simulink model "th_discrete_time_integrator"  (R2020b)
settings: Solver=VariableStepAuto  StartTime=0.0  StopTime=6  RelTol=1e-3
values from neighbouring files (symbols this model uses):
  parInitCondInitVal = 0.0    [dd_discrete_time_integrator.sldd]
  parInpInitVal = 0.0    [dd_discrete_time_integrator.sldd]
  parIntgGain = 1.0    [dd_discrete_time_integrator.sldd]
  parLowLimInitVal = 0.0    [dd_discrete_time_integrator.sldd]
  parOutpDataTypeInhrFlag = 1    [dd_discrete_time_integrator.sldd]
  parRsetCondInitVal = 0.0    [dd_discrete_time_integrator.sldd]
  parSampTime = 0.01    [dd_discrete_time_integrator.sldd]
  parSatFlag = 0.0    [dd_discrete_time_integrator.sldd]
  parTestProcInitCondIndx = 0.0    [dd_discrete_time_integrator.sldd]
  parTestProcInpIndx = 1.0    [dd_discrete_time_integrator.sldd]
  parTestProcLowLimIndx = 0.0    [dd_discrete_time_integrator.sldd]
  parTestProcRsetCondIndx = 0.0    [dd_discrete_time_integrator.sldd]
  parTestProcUpLimIndx = 0.0    [dd_discrete_time_integrator.sldd]
  parUpLimInitVal = 0.0    [dd_discrete_time_integrator.sldd]
undefined symbols (not defined in the file or in its folder): DiscIntNeverNeededParam
settings Model: DataDictionary=dd_discrete_time_integrator.sldd  Creator=CAV2OFO  LastModifiedBy=CAV2OFO
settings DebuggingCC: SFUnusedDataAndEventsDiag=none

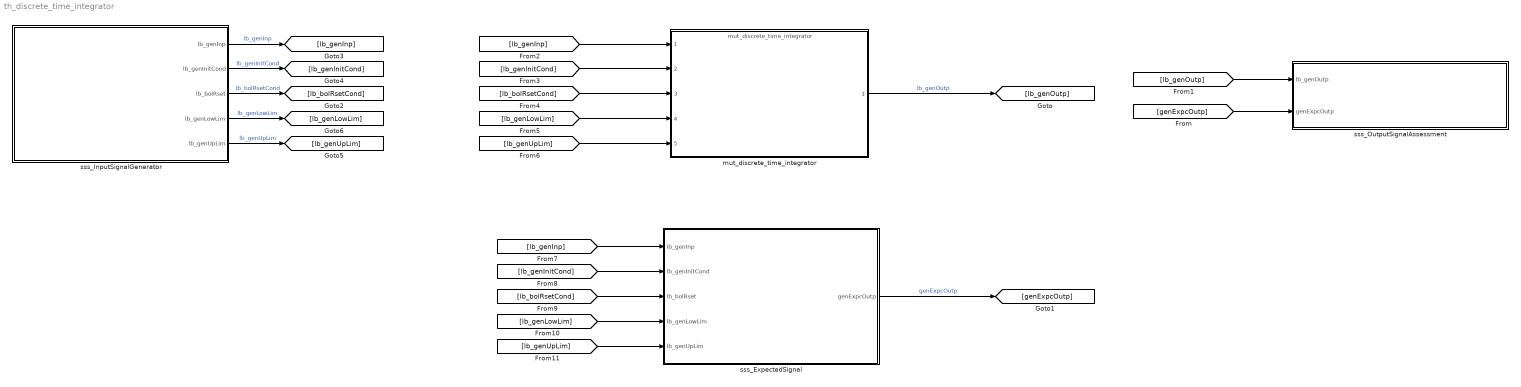
== system th_discrete_time_integrator ==
  mut_discrete_time_integrator : ModelReference  ModelNameDialog=mut_discrete_time_integrator  SimulationMode=Normal  ModelReferenceVersion=1.22
  sss_ExpectedSignal : Subsystem
  sss_InputSignalGenerator : Subsystem
  sss_OutputSignalAssessment : Subsystem
  wires:
  [lb_genUpLim] -> mut_discrete_time_integrator/5
  [lb_genInitCond] -> sss_ExpectedSignal/2(lb_genInitCond)
  sss_InputSignalGenerator/1(lb_genInp) -> [lb_genInp]  "lb_genInp"
  mut_discrete_time_integrator/1 -> [lb_genOutp]  "lb_genOutp"
  [lb_bolRsetCond] -> sss_ExpectedSignal/3(lb_bolRset)
  [lb_genOutp] -> sss_OutputSignalAssessment/1(lb_genOutp)
  [lb_genInitCond] -> mut_discrete_time_integrator/2
  sss_InputSignalGenerator/5(lb_genUpLim) -> [lb_genUpLim]  "lb_genUpLim"
  [genExpcOutp] -> sss_OutputSignalAssessment/2(genExpcOutp)
  [lb_genLowLim] -> sss_ExpectedSignal/4(lb_genLowLim)
  sss_InputSignalGenerator/4(lb_genLowLim) -> [lb_genLowLim]  "lb_genLowLim"
  [lb_bolRsetCond] -> mut_discrete_time_integrator/3
  sss_InputSignalGenerator/2(lb_genInitCond) -> [lb_genInitCond]  "lb_genInitCond"
  [lb_genUpLim] -> sss_ExpectedSignal/5(lb_genUpLim)
  sss_InputSignalGenerator/3(lb_bolRset) -> [lb_bolRsetCond]  "lb_bolRsetCond"
  sss_ExpectedSignal/1(genExpcOutp) -> [genExpcOutp]  "genExpcOutp"
  [lb_genInp] -> sss_ExpectedSignal/1(lb_genInp)
  [lb_genInp] -> mut_discrete_time_integrator/1
  [lb_genLowLim] -> mut_discrete_time_integrator/4

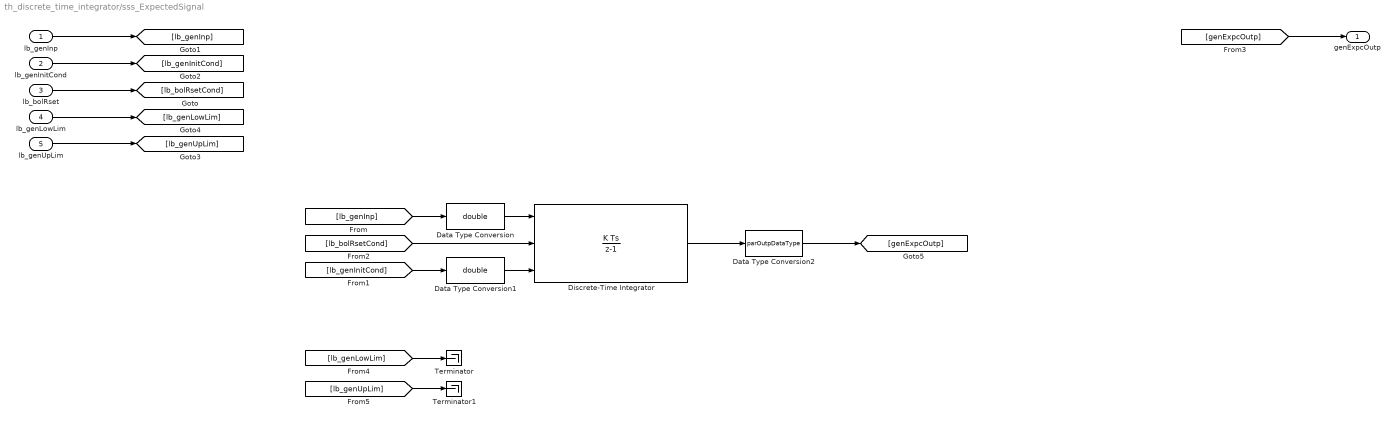
== system th_discrete_time_integrator/sss_ExpectedSignal ==
  lb_genInp : Inport
  lb_genInitCond : Inport  Port=2
  lb_bolRset : Inport  Port=3
  lb_genLowLim : Inport  Port=4
  lb_genUpLim : Inport  Port=5
  Data Type Conversion : DataTypeConversion  OutDataTypeStr=double
  Data Type Conversion1 : DataTypeConversion  OutDataTypeStr=double
  Data Type Conversion2 : DataTypeConversion  OutDataTypeStr=parOutpDataType
  Discrete-Time Integrator : DiscreteIntegrator  gainval=double(parIntgGain)  ExternalReset=level  InitialConditionSource=external  SampleTime=double(parSampTime)  LimitOutput=on  UpperSaturationLimit=double(parUpLimInitVal)  LowerSaturationLimit=double(parLowLimInitVal)  ICPrevOutput=DiscIntNeverNeededParam  ICPrevScaledInput=DiscIntNeverNeededParam
  Terminator : Terminator
  Terminator1 : Terminator
  genExpcOutp : Outport
  wires:
  lb_bolRset/1 -> [lb_bolRsetCond]
  lb_genInp/1 -> [lb_genInp]
  lb_genInitCond/1 -> [lb_genInitCond]
  lb_genLowLim/1 -> [lb_genLowLim]
  lb_genUpLim/1 -> [lb_genUpLim]
  [lb_bolRsetCond] -> Discrete-Time Integrator/2
  [genExpcOutp] -> genExpcOutp/1
  Discrete-Time Integrator/1 -> Data Type Conversion2/1
  [lb_genInitCond] -> Data Type Conversion1/1
  [lb_genInp] -> Data Type Conversion/1
  Data Type Conversion1/1 -> Discrete-Time Integrator/3
  Data Type Conversion2/1 -> [genExpcOutp]
  Data Type Conversion/1 -> Discrete-Time Integrator/1
  [lb_genLowLim] -> Terminator/1
  [lb_genUpLim] -> Terminator1/1

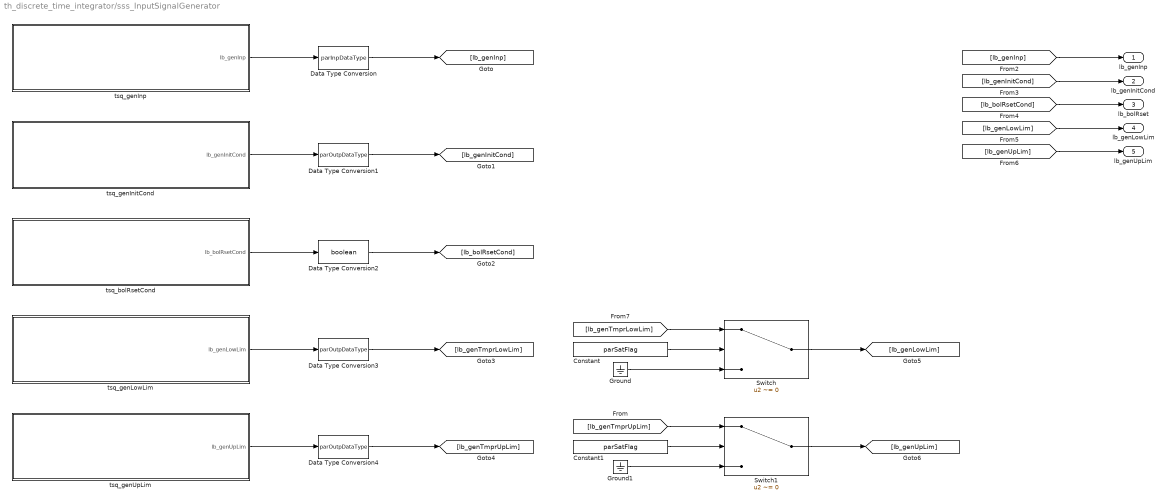
== system th_discrete_time_integrator/sss_InputSignalGenerator ==
  Constant : Constant  Value=parSatFlag
  Constant1 : Constant  Value=parSatFlag
  Data Type Conversion : DataTypeConversion  OutDataTypeStr=parInpDataType
  Data Type Conversion1 : DataTypeConversion  OutDataTypeStr=parOutpDataType
  Data Type Conversion2 : DataTypeConversion  OutDataTypeStr=boolean
  Data Type Conversion3 : DataTypeConversion  OutDataTypeStr=parOutpDataType
  Data Type Conversion4 : DataTypeConversion  OutDataTypeStr=parOutpDataType
  Ground : Ground
  Ground1 : Ground
  Switch : Switch  Criteria=u2 ~= 0
  Switch1 : Switch  Criteria=u2 ~= 0
  tsq_bolRsetCond : Test Sequence  TreatAsAtomicUnit=on
  tsq_genInitCond : Test Sequence  TreatAsAtomicUnit=on
  tsq_genInp : Test Sequence  TreatAsAtomicUnit=on
  tsq_genLowLim : Test Sequence  TreatAsAtomicUnit=on
  tsq_genUpLim : Test Sequence  TreatAsAtomicUnit=on
  lb_genInp : Outport
  lb_genInitCond : Outport  Port=2
  lb_bolRset : Outport  Port=3
  lb_genLowLim : Outport  Port=4
  lb_genUpLim : Outport  Port=5
  wires:
  [lb_genInitCond] -> lb_genInitCond/1
  [lb_genInp] -> lb_genInp/1
  [lb_bolRsetCond] -> lb_bolRset/1
  [lb_genLowLim] -> lb_genLowLim/1
  [lb_genUpLim] -> lb_genUpLim/1
  tsq_genInp/1(lb_genInp) -> Data Type Conversion/1
  Data Type Conversion/1 -> [lb_genInp]
  Data Type Conversion1/1 -> [lb_genInitCond]
  tsq_genInitCond/1(lb_genInitCond) -> Data Type Conversion1/1
  Data Type Conversion2/1 -> [lb_bolRsetCond]
  tsq_bolRsetCond/1(lb_bolRsetCond) -> Data Type Conversion2/1
  Data Type Conversion3/1 -> [lb_genTmprLowLim]
  tsq_genLowLim/1(lb_genLowLim) -> Data Type Conversion3/1
  Data Type Conversion4/1 -> [lb_genTmprUpLim]
  tsq_genUpLim/1(lb_genUpLim) -> Data Type Conversion4/1
  Constant/1 -> Switch/2
  [lb_genTmprLowLim] -> Switch/1
  Ground/1 -> Switch/3
  [lb_genTmprUpLim] -> Switch1/1
  Constant1/1 -> Switch1/2
  Ground1/1 -> Switch1/3
  Switch/1 -> [lb_genLowLim]
  Switch1/1 -> [lb_genUpLim]

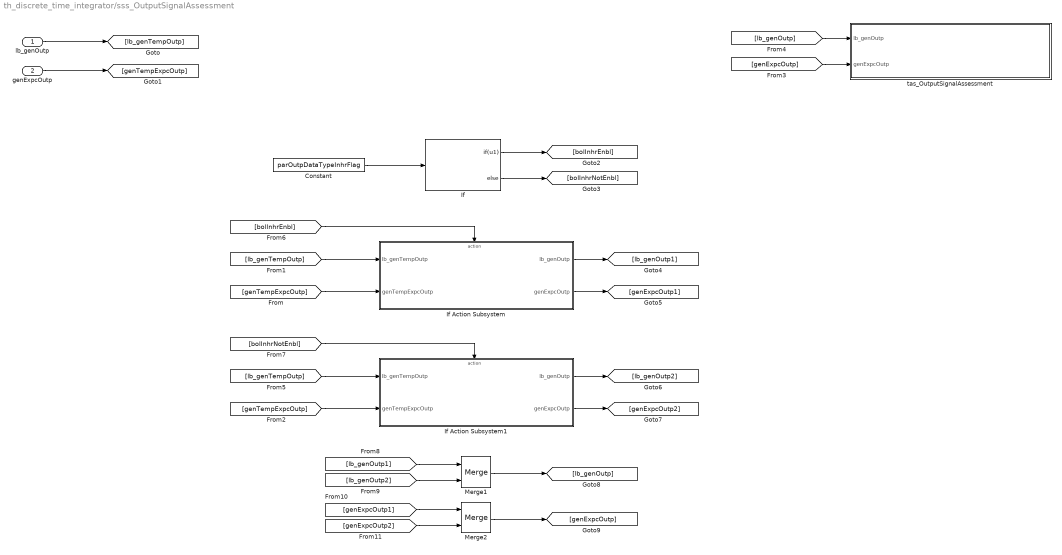
== system th_discrete_time_integrator/sss_OutputSignalAssessment ==
  lb_genOutp : Inport
  genExpcOutp : Inport  Port=2
  Constant : Constant  Value=parOutpDataTypeInhrFlag
  If : If  IfExpression=u1
  If Action Subsystem : Subsystem  TreatAsAtomicUnit=on
  If Action Subsystem1 : Subsystem  TreatAsAtomicUnit=on
  Merge1 : Merge
  Merge2 : Merge
  tas_OutputSignalAssessment : Test Sequence  TreatAsAtomicUnit=on
  wires:
  [lb_genOutp] -> tas_OutputSignalAssessment/1(lb_genOutp)
  [genExpcOutp] -> tas_OutputSignalAssessment/2(genExpcOutp)
  lb_genOutp/1 -> [lb_genTempOutp]
  genExpcOutp/1 -> [genTempExpcOutp]
  Constant/1 -> If/1
  [lb_genTempOutp] -> If Action Subsystem/1(lb_genTempOutp)
  [genTempExpcOutp] -> If Action Subsystem/2(genTempExpcOutp)
  [genTempExpcOutp] -> If Action Subsystem1/2(genTempExpcOutp)
  [lb_genTempOutp] -> If Action Subsystem1/1(lb_genTempOutp)
  If/1 -> [bolInhrEnbl]
  [bolInhrEnbl] -> If Action Subsystem/Action
  If/2 -> [bolInhrNotEnbl]
  [bolInhrNotEnbl] -> If Action Subsystem1/Action
  If Action Subsystem/2(genExpcOutp) -> [genExpcOutp1]
  If Action Subsystem/1(lb_genOutp) -> [lb_genOutp1]
  If Action Subsystem1/1(lb_genOutp) -> [lb_genOutp2]
  If Action Subsystem1/2(genExpcOutp) -> [genExpcOutp2]
  [lb_genOutp1] -> Merge1/1
  [lb_genOutp2] -> Merge1/2
  [genExpcOutp1] -> Merge2/1
  [genExpcOutp2] -> Merge2/2
  Merge1/1 -> [lb_genOutp]
  Merge2/1 -> [genExpcOutp]

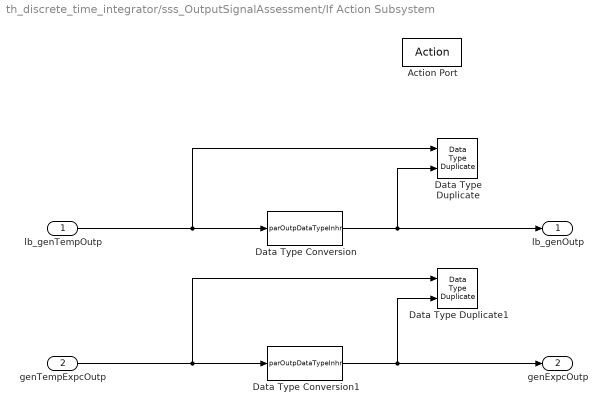
== system th_discrete_time_integrator/sss_OutputSignalAssessment/If Action Subsystem ==
  lb_genTempOutp : Inport
  genTempExpcOutp : Inport  Port=2
  Action Port : ActionPort  ActionPortLabel=if(u1)
  Data Type Duplicate : DataTypeDuplicate
  Data Type Duplicate1 : DataTypeDuplicate
  Data Type Conversion : DataTypeConversion  OutDataTypeStr=parOutpDataTypeInhr
  Data Type Conversion1 : DataTypeConversion  OutDataTypeStr=parOutpDataTypeInhr
  lb_genOutp : Outport
  genExpcOutp : Outport  Port=2
  wires:
  lb_genTempOutp/1 -> Data Type Duplicate/1, Data Type Conversion/1
  Data Type Conversion/1 -> Data Type Duplicate/2, lb_genOutp/1
  Data Type Conversion1/1 -> Data Type Duplicate1/2, genExpcOutp/1
  genTempExpcOutp/1 -> Data Type Duplicate1/1, Data Type Conversion1/1

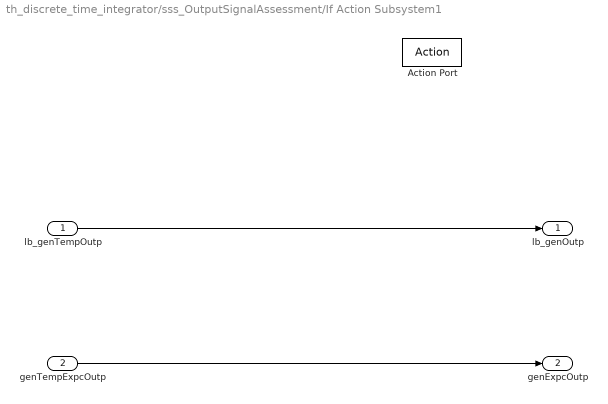
== system th_discrete_time_integrator/sss_OutputSignalAssessment/If Action Subsystem1 ==
  lb_genTempOutp : Inport
  genTempExpcOutp : Inport  Port=2
  Action Port : ActionPort  ActionPortLabel=else
  lb_genOutp : Outport
  genExpcOutp : Outport  Port=2
  wires:
  lb_genTempOutp/1 -> lb_genOutp/1
  genTempExpcOutp/1 -> genExpcOutp/1

== stateflow chart th_discrete_time_integrator/sss_OutputSignalAssessment/tas_OutputSignalAssessment ==
  settings: stateMachineType=SIMPLIFIED_MACHINE
  state verify
    if genExpcOutp == 0
    error = 0;
    else
    error = abs(double((lb_genOutp - genExpcOutp)/genExpcOutp));
    end
    verify(error <= parTestTol,'The actual and expected output matches');
  (default) -> verify
  data: lb_genOutp input; genExpcOutp input; parTestTol parameter; error local

== stateflow chart th_discrete_time_integrator/sss_InputSignalGenerator/tsq_genInitCond ==
  settings: stateMachineType=SIMPLIFIED_MACHINE
  state Init
    lb_genInitCond = double(parInitCondInitVal);
  (default) -> Init
  data: lb_genInitCond output; parInitCondInitVal parameter; parTestProcInitCondIndx parameter

== stateflow chart th_discrete_time_integrator/sss_InputSignalGenerator/tsq_bolRsetCond ==
  settings: stateMachineType=SIMPLIFIED_MACHINE
  state Init
    lb_bolRsetCond = parRsetCondInitVal;
  (default) -> Init
  data: lb_bolRsetCond output boolean; parRsetCondInitVal parameter; parTestProcRsetCondIndx parameter

== stateflow chart th_discrete_time_integrator/sss_InputSignalGenerator/tsq_genInp ==
  settings: stateMachineType=SIMPLIFIED_MACHINE
  state Init
    lb_genInp = double(parInpInitVal);
  state TestProcedure_1
    state TestProcedure_1_ramp
      lb_genInp = double(parInpInitVal) + ramp(et);
    state TestProcedure_1_end
    (default) -> TestProcedure_1_ramp
    TestProcedure_1_ramp -> TestProcedure_1_end : [
        | after(5,sec)
        | ]
  (default) -> Init
  Init -> TestProcedure_1 : [
      | parTestProcInpIndx == 1
      | ]
  data: lb_genInp output double; parTestProcInpIndx parameter; parInpInitVal parameter

== stateflow chart th_discrete_time_integrator/sss_InputSignalGenerator/tsq_genLowLim ==
  settings: stateMachineType=SIMPLIFIED_MACHINE
  state Init
    lb_genLowLim = double(parLowLimInitVal);
  (default) -> Init
  data: lb_genLowLim output; parLowLimInitVal parameter; parTestProcLowLimIndx parameter

== stateflow chart th_discrete_time_integrator/sss_InputSignalGenerator/tsq_genUpLim ==
  settings: stateMachineType=SIMPLIFIED_MACHINE
  state Init
    lb_genUpLim = double(parUpLimInitVal);
  (default) -> Init
  data: lb_genUpLim output; parUpLimInitVal parameter; parTestProcUpLimIndx parameter
